simulink model "PWM_motor"  (R2014a)
settings: Solver=ode23s  StartTime=0.0  StopTime=2.5  MaxStep=2e-6  RelTol=1e-3  AbsTol=.01
libraries: powerlib x13, simulink x2, powerlib_meascontrol x2
settings Model: CovSFcnEnable=on  Creator=lenovo  LastModifiedBy=DELL
settings SolverCC: ZeroCrossAlgorithm=Adaptive
settings DataIOCC: SignalLoggingSaveFormat=ModelDataLogs
settings OptimizationCC: InitFltsAndDblsToZero=on
settings DebuggingCC: SaveWithParameterizedLinksMsg=none  UnderspecifiedInitializationDetection=Classic  SignalResolutionControl=TryResolveAllWithWarning  MaxConsecutiveZCsMsg=none  MultiTaskDSMMsg=warning  MultiTaskCondExecSysMsg=none  FcnCallInpInsideContextMsg=EnableAllAsWarning  FrameProcessingCompatibilityMsg=error
settings GRTTargetCC: TargetFcnLib=ansi_tfl_tmw.mat  CombineOutputUpdateFcns=off  GRTInterface=on
settings ConfigurationSet: Description=Simscape Multibody

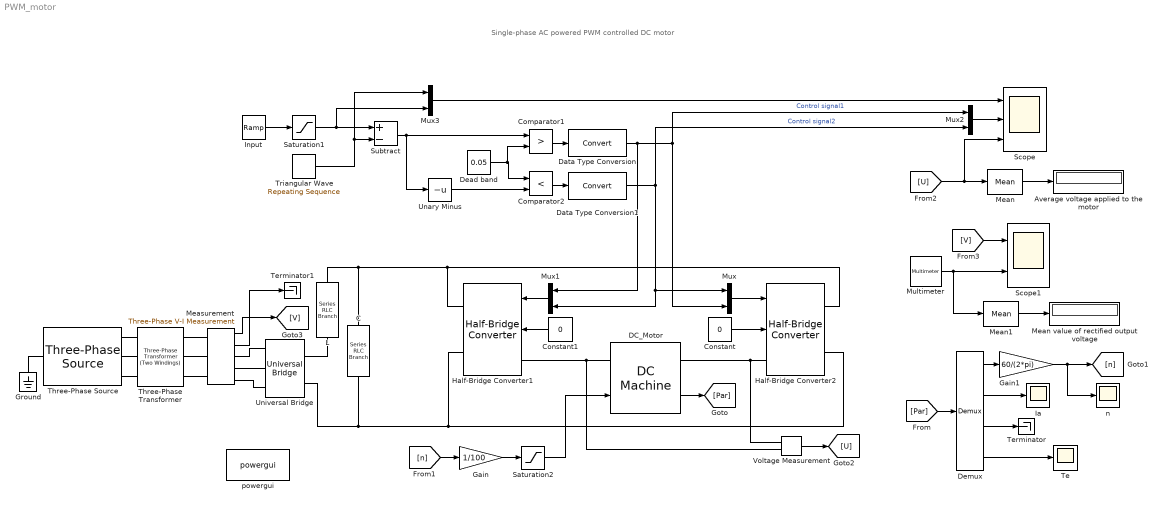
== system PWM_motor ==
  note: Single-phase AC powered PWM controlled DC motor
  Average voltage applied to the motor : Display
  C : powerlib/Elements/Series RLC Branch  LConnTagsString=__new0  RConnTagsString=__new0  BranchType=C  Resistance=50  Inductance=30e-3  SetiL0=off  InitialCurrent=0  Capacitance=5000e-6  Setx0=on  InitialVoltage=27  Measurements=Branch voltage
  Comparator1 : RelationalOperator  Operator=>  OutDataTypeStr=boolean
  Comparator2 : RelationalOperator  Operator=<  OutDataTypeStr=boolean
  Constant : Constant  Value=0
  Constant1 : Constant  Value=0
  DC_Motor : powerlib/Machines/DC Machine  PresetModel=No  MechanicalLoad=Torque TL  FieldType=Permanent magnet  ShowDetailedParameters=on  MeasurementBus=off  RLa="[ 4.767  1.2e-3]"  RLf="[ 183.333  0]"  Laf=2.400  MachineConstant=Torque constant (N.m/A)  Ke=1.8  Kt=0.5  J=1e-3  Bm=0  Tf=0  w0=0  Ifinit=1  TsPowergui=0  TsBlock=-1
      settings: AttributesFormatString=\n
  Data Type Conversion : DataTypeConversion
  Data Type Conversion1 : DataTypeConversion
  Dead band : Constant  Value=0.05
  Demux : Demux
      settings: DisplayOption=none
  Gain : Gain  Gain=1/100
  Gain1 : Gain  Gain=60/(2*pi)
  Ground : powerlib/Elements/Ground  LConnTagsString=a
  Half-Bridge Converter1 : powerlib/Power Electronics/Half-Bridge Converter  ModelType=Switching devices  Ron=1e-3  Rs=1e6  Cs=inf  Vforward=[0,0]  Ron_Diode=1e-3  Rs_Diode=1e6  Cs_Diode=inf  Vf_Diode=1e-3  Rs_CurrentSource=inf
  Half-Bridge Converter2 : powerlib/Power Electronics/Half-Bridge Converter  ModelType=Switching devices  Ron=1e-3  Rs=1e6  Cs=inf  Vforward=[0,0]  Ron_Diode=1e-3  Rs_Diode=1e6  Cs_Diode=inf  Vf_Diode=1e-3  Rs_CurrentSource=inf
  Ia : Scope
      settings: TimeRange=auto  MaxDataPoints=5000  SaveToWorkspace=off  SaveName=ScopeData2  YMin=-1.40309  YMax=2.62602  SampleTime=-1
  Input : simulink/Sources/Ramp  slope=0.4  start=0  X0=0
      settings: AttributesFormatString=slope=%<slope>
  L : powerlib/Elements/Series RLC Branch  LConnTagsString=__new0  RConnTagsString=__new0  BranchType=L  Resistance=50  Inductance=200e-6  SetiL0=off  InitialCurrent=0  Capacitance=1e-6  Setx0=off  InitialVoltage=0  Measurements=None
  Mean : powerlib_meascontrol/Measurements/Mean  Freq=50  Vinit=0  Ts=0  treatSBRowAsCol=off
  Mean value of rectified output voltage : Display
  Mean1 : powerlib_meascontrol/Measurements/Mean  Freq=50  Vinit=0  Ts=0  treatSBRowAsCol=off
  Measurement : powerlib/Measurements/Three-Phase V-I Measurement  VoltageMeasurement=phase-to-phase  SetLabelV=off  LabelV=Vabc  Vpu=off  VpuLL=off  CurrentMeasurement=yes  SetLabelI=off  LabelI=Iabc  Ipu=off  Pbase=100e6  Vbase=500e3  OutputType=Complex  PhasorSimulation=off  PSBequivalent=0
  Multimeter : powerlib/Measurements/Multimeter  PhasorSimulation=off  OutputType=Complex  sel=1  L=1  Gain=1  yselected={'Ub: C'};  PSBOutputType=1  PSBequivalent=0  AxesSetting=[0,0.1,-100,100]  Display=0  SavedBlockNames=-11
  Mux{,1..3} (4 alike) : Mux  Inputs=2
  Saturation1 : Saturate  UpperLimit=0.8  LowerLimit=0
      settings: AttributesFormatString=UpperLimit=%<UpperLimit>
  Saturation2 : Saturate  UpperLimit=1  LowerLimit=0
      settings: AttributesFormatString=UpperLimit=%<UpperLimit>
  Scope : Scope  NumInputPorts=3
      settings: TimeRange=auto  ShowLegends=on  MaxDataPoints=5000  SaveToWorkspace=off  SaveName=ScopeData  YMin=-1.24999~-0.125~-33.74989  YMax=1.24999~1.125~33.74905  SampleTime=-1
  Scope1 : Scope  NumInputPorts=2
      settings: TimeRange=auto  ShowLegends=on  MaxDataPoints=5000  SaveToWorkspace=off  SaveName=ScopeData4  YMin=-385.45727~19.85029  YMax=385.45796~20.14555  SampleTime=-1
  Subtract : Sum  Inputs=+-
  Te : Scope
      settings: TimeRange=auto  MaxDataPoints=5000  SaveToWorkspace=off  SaveName=ScopeData3  YMin=-0.70154  YMax=1.31301  SampleTime=-1
  Terminator : Terminator
  Terminator1 : Terminator
  Three-Phase Transformer : powerlib/Elements/Three-Phase Transformer (Two Windings)  Winding1Connection=Y  Winding2Connection=Yg  CoreType=Three single-phase transformers  SetSaturation=off  Hysteresis=off  DataFile='hysteresis'  SetInitialFlux=off  Measurements=None  UNITS=pu  NominalPower=[ 250e6 , 50 ]  Winding1=[ 380e3 , 0.002 , 0.08 ]  Winding2=[ 15e3 , 0.002 , 0.08 ]  Rm=500  Lm=500  L0=0.5  Saturation=[ 0,0 ; 0.0024,1.2 ; 1.0,1.52 ]  InitialFluxes=[ 0.8 , -0.8 , 0.7 ]  BreakLoop=off  DiscreteSolver=Trapezoidal iterative  DataType=off  TransfoNumber=1
      settings: AttributesFormatString=|
      | Winding1=%<Winding1>
      | Winding2=%<Winding2>
  Three-Phase Source : powerlib/Electrical Sources/Three-Phase Source  InternalConnection=Yn  VoltagePhases=off  Voltage=380  PhaseAngle=0  Voltage_phases=[25e3 25e3 25e3]/sqrt(3)  PhaseAngles_phases=[0 -120 +120]  Frequency=50  NonIdealSource=on  SpecifyImpedance=off  Resistance=0  Inductance=0  ShortCircuitLevel=100e6  BaseVoltage=100*sqrt(3/2)  XRratio=7  BusType=swing  Pref=10e3  Qref=0  Prefabc=[10e3, 10e3, 10e3]  Qrefabc=[0, 0, 0]  Qmin=-inf  Qmax=inf
      settings: AttributesFormatString=Voltage=%<Voltage>
  Triangular Wave : simulink/Sources/Repeating Sequence  rep_seq_t=[0 2.5e-5 7.5e-5 1e-4]  rep_seq_y=[0 1 -1 0]
  Unary Minus : UnaryMinus
  Universal Bridge : powerlib/Power Electronics/Universal Bridge  Arms=3  SnubberResistance=1e5  SnubberCapacitance=inf  Device=Diodes  Ron=1e-3  Lon=0  ForwardVoltages="[  0  0  ]"  ForwardVoltage=0  GTOparameters=[ 10e-6 , 20e-6 ]  IGBTparameters=[ 1e-6 , 2e-6 ]  Measurements=None  Measurements_2=None  converterType=Rectifier
  Voltage Measurement : powerlib/Measurements/Voltage Measurement  PhasorSimulation=off  OutputType=Complex  PSBequivalent=0
  n : Scope
      settings: TimeRange=auto  MaxDataPoints=5000  SaveToWorkspace=off  YMin=115.13531  YMax=115.70828  SampleTime=-1
  powergui : powerlib/powergui  Priority=1  SimulationMode=Continuous  SampleTime=50e-6  frequency=60  Iterations=50  frequencyindice=0  Pbase=100e6  ErrMax=1e-4  UnitsV=kV  UnitsW=MW  buscounter=0  FunctionMessages=off  echomessages=off  EnableUseOfTLC=off  CurrentSourceSwitches=off  DisableSnubberDevices=off  DisableRonSwitches=off  DisableVfSwitches=off  DisplayEquations=off  AutomaticDiscreteSolvers=off  SolverType=Tustin/Backward Euler (TBE)  Interpol=off  ExternalGateDelay=off  methode=off  Ts=100  x0status=blocks  SPID=on  SwTol=0  HookPort=off  NonlinearTolerance=1e-4  nMaxIteration=100  ContinueOnMaxIteration=off  RestoreLinks=warning  ResistiveCurrentMeasurement=off  Frange=[0:2:500]  Ylog=off  Xlog=on  ShowGrid=off  save=off  variable=ZData  structure=ScopeData  ZoomFFT=off  StartTime=0.01  cycles=5  DisplayStyle=1  fundamental=3000  FreqAxis=off  MaxFrequency=60000  frequencyindicesteady=1  RmsSteady=1  display=off
  wires:
  Comparator1/1 -> Data Type Conversion/1
  Input/1 -> Saturation1/1
  Data Type Conversion/1 -> Mux1/1, Mux/2, Mux2/1  "Control signal1"
  Data Type Conversion1/1 -> Mux/1, Mux1/2, Mux2/2  "Control signal2"
  Mux1/1 -> Half-Bridge Converter1/1
  Mux/1 -> Half-Bridge Converter2/1
  Constant/1 -> Half-Bridge Converter2/2
  Constant1/1 -> Half-Bridge Converter1/2
  Demux/3 -> Terminator/1
  Demux/4 -> Te/1
  Demux/2 -> Ia/1
  Demux/1 -> Gain1/1
  DC_Motor/1 -> [Par]
  [Par] -> Demux/1
  Gain1/1 -> [n], n/1
  Voltage Measurement/1 -> [U]
  Mean/1 -> Average voltage applied to the motor/1
  Gain/1 -> Saturation2/1
  [n] -> Gain/1
  Saturation2/1 -> DC_Motor/1
  Measurement/2 -> Terminator1/1
  Measurement/1 -> [V]
  [V] -> Scope1/1
  Multimeter/1 -> Mean1/1, Scope1/2
  Mean1/1 -> Mean value of rectified output voltage/1
  Saturation1/1 -> Mux3/2, Subtract/1
  Triangular Wave/1 -> Mux3/1, Subtract/2
  Dead band/1 -> Comparator1/2, Comparator2/1
  Subtract/1 -> Unary Minus/1, Comparator1/1
  Unary Minus/1 -> Comparator2/2
  Comparator2/1 -> Data Type Conversion1/1
  Mux2/1 -> Scope/2
  Mux3/1 -> Scope/1
  [U] -> Mean/1, Scope/3
  connections:
  Half-Bridge Converter2/LConn1 -- Voltage Measurement/LConn2 -- DC_Motor/RConn1
  Half-Bridge Converter1/LConn1 -- Voltage Measurement/LConn1 -- DC_Motor/LConn1
  C/LConn1 -- L/RConn1 -- Half-Bridge Converter2/RConn1 -- Half-Bridge Converter1/RConn1
  C/RConn1 -- Universal Bridge/RConn2 -- Half-Bridge Converter2/RConn2 -- Half-Bridge Converter1/RConn2
  Three-Phase Source/RConn2 -- Three-Phase Transformer/LConn2
  Three-Phase Source/LConn1 -- Ground/LConn1
  Three-Phase Transformer/LConn3 -- Three-Phase Source/RConn3
  Three-Phase Transformer/LConn1 -- Three-Phase Source/RConn1
  Measurement/LConn1 -- Three-Phase Transformer/RConn1
  Measurement/LConn2 -- Three-Phase Transformer/RConn2
  Measurement/LConn3 -- Three-Phase Transformer/RConn3
  Universal Bridge/LConn2 -- Measurement/RConn2
  Measurement/RConn1 -- Universal Bridge/LConn1
  Measurement/RConn3 -- Universal Bridge/LConn3
  Universal Bridge/RConn1 -- L/LConn1
